simulink model "GILBERT1FINAL"  (R2023a)
settings: Solver=VariableStepAuto  StartTime=0.0  StopTime=10.0  RelTol=1e-3
undefined symbols (not defined in the file): Acid, Lead
libraries: spsSeriesRLCBranchLib x5, spsBreakerLib x4, spsBatteryLib x3, spsPVArrayLib x1, spsParallelRLCBranchLib x1, spspowerguiLib x1
settings Model: Creator=InnoTech  LastModifiedBy=Karim

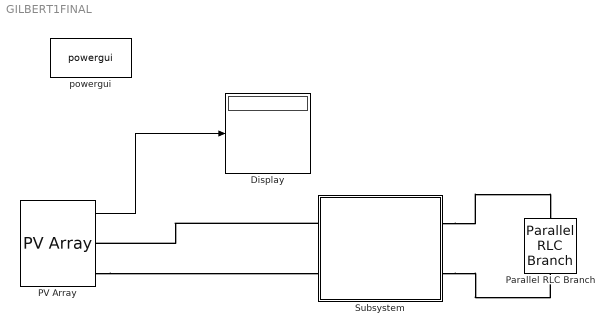
== system GILBERT1FINAL ==
  Display : Display
  PV Array : spsPVArrayLib/PV Array  Npar=40  Nser=10  PlotType=array @ 1000 W/m2 & specified temperatures  S_vec="[ 1000  500  100 ]"  Temp_C_vec="[ 45 25  ]"  ModuleName=User-defined  PlotWhenSelected=off  Pm=213.15  Ncell=60  Voc=36.3  Isc=7.84  Vm=29  Im=7.35  beta_Voc_pc=-0.36099  alpha_Isc_pc=0.102  beta_Voc=-0.13104  alpha_Isc=0.0079968  IL=7.8654  I0=2.9273e-10  nI=0.98119  Rsh=313.0553  Rs=0.39381  RobustModel=off  RobustCellTemperature=313.3991  BAL=on  Tc=1e-6  Tfilter=5e-5
  Parallel RLC Branch : spsParallelRLCBranchLib/Parallel RLC Branch  LConnTagsString=a  RConnTagsString=__new0  BranchType=RLC  Resistance=1  Inductance=1e-3  SetiL0=off  InitialCurrent=0  Capacitance=1e-6  Setx0=off  InitialVoltage=0  Measurements=None
  Subsystem : Subsystem
  powergui : spspowerguiLib/powergui  Priority=1  SimulationMode=Discrete  SampleTime=50e-6  frequency=60  Iterations=50  frequencyindice=0  Pbase=100e6  ErrMax=1e-4  UnitsV=kV  UnitsW=MW  buscounter=0  FunctionMessages=off  echomessages=off  EnableUseOfTLC=off  CurrentSourceSwitches=off  DisableSnubberDevices=off  DisableRonSwitches=off  DisableVfSwitches=off  DisplayEquations=off  AutomaticDiscreteSolvers=off  SolverType=Tustin/Backward Euler (TBE)  Interpol=off  ExternalGateDelay=off  methode=off  Ts=100  x0status=blocks  SPID=on  SwTol=0  HookPort=off  NonlinearTolerance=1e-4  nMaxIteration=100  ContinueOnMaxIteration=off  RestoreLinks=warning  ResistiveCurrentMeasurement=off  Frange=[0:2:500]  Ylog=off  Xlog=on  ShowGrid=off  save=off  variable=ZData  structure=0  ZoomFFT=off  StartTime=0.0  cycles=1  DisplayStyle=1  fundamental=60  FreqAxis=off  MaxFrequency=1000  frequencyindicesteady=1  RmsSteady=1  display=off
  wires:
  PV Array/1 -> Display/1
  connections:
  Subsystem/LConn1 -- PV Array/RConn1
  PV Array/RConn2 -- Subsystem/LConn2
  Subsystem/RConn1 -- Parallel RLC Branch/LConn1
  Subsystem/RConn2 -- Parallel RLC Branch/RConn1

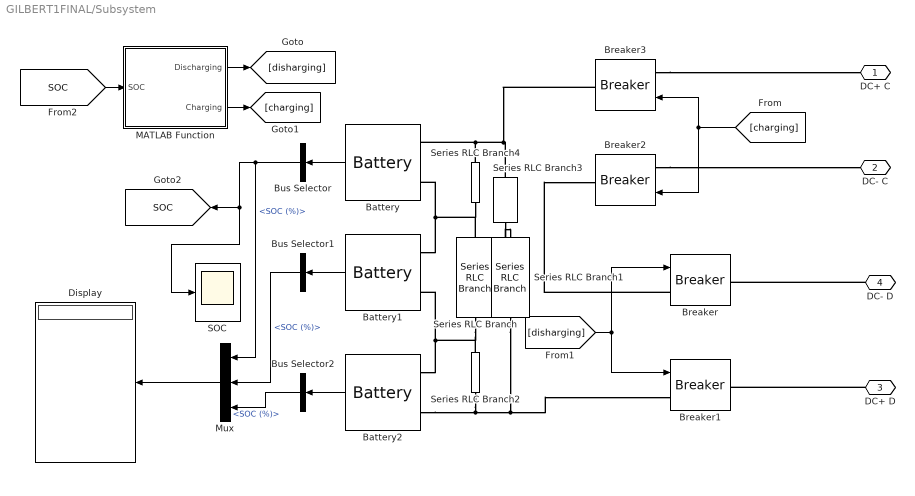
== system GILBERT1FINAL/Subsystem ==
  Battery : spsBatteryLib/Battery  BatType=Lead-Acid  NomV=12*50  NomQ=141.65  SOC=50  Batt_Tr=30  PresetModel=on  MaxQ=147.5521  MinV=450  FullV=653.2895  Dis_rate=28.33  R=0.042358  Normal_OP=43.9508  expZone="[610.8553     0.4721667]"
  Battery1 : spsBatteryLib/Battery  BatType=Lead-Acid  NomV=12*50  NomQ=141.65  SOC=50  Batt_Tr=30  PresetModel=on  MaxQ=147.5521  MinV=450  FullV=653.2895  Dis_rate=28.33  R=0.042358  Normal_OP=43.9508  expZone="[610.8553     0.4721667]"
  Battery2 : spsBatteryLib/Battery  BatType=Lead-Acid  NomV=12*50  NomQ=141.65  SOC=50  Batt_Tr=30  PresetModel=on  MaxQ=147.5521  MinV=450  FullV=653.2895  Dis_rate=28.33  R=0.042358  Normal_OP=43.9508  expZone="[610.8553     0.4721667]"
  Breaker{,1..3} (4 alike) : spsBreakerLib/Breaker  InitialState=0  SwitchingTimes="[1/60  5/60]"  External=on  BreakerResistance=0.01  SnubberResistance=1e6  SnubberCapacitance=inf  Measurements=None  MoreParameters=on  NoBreakLoop=off
  Bus Selector : BusSelector  OutputSignals=SOC (%)
  Bus Selector1 : BusSelector  OutputSignals=SOC (%)
  Bus Selector2 : BusSelector  OutputSignals=SOC (%)
  Display : Display
  MATLAB Function : MATLAB Function  TreatAsAtomicUnit=on
  Mux : Mux  Inputs=3
  SOC : Scope
  Series RLC Branch : spsSeriesRLCBranchLib/Series RLC Branch  LConnTagsString=__new0  RConnTagsString=__new0  BranchType=R  Resistance=100  Inductance=1e-3  SetiL0=off  InitialCurrent=0  Capacitance=1e-6  Setx0=off  InitialVoltage=0  Measurements=None
  Series RLC Branch1 : spsSeriesRLCBranchLib/Series RLC Branch  LConnTagsString=__new0  RConnTagsString=__new0  BranchType=C  Resistance=100  Inductance=1e-3  SetiL0=off  InitialCurrent=0  Capacitance=1e-6  Setx0=off  InitialVoltage=0  Measurements=None
  Series RLC Branch2 : spsSeriesRLCBranchLib/Series RLC Branch  LConnTagsString=__new0  RConnTagsString=__new0  BranchType=L  Resistance=100  Inductance=1e-3  SetiL0=off  InitialCurrent=0  Capacitance=1e-6  Setx0=off  InitialVoltage=0  Measurements=None
  Series RLC Branch3 : spsSeriesRLCBranchLib/Series RLC Branch  LConnTagsString=__new0  RConnTagsString=__new0  BranchType=R  Resistance=1  Inductance=1e-3  SetiL0=off  InitialCurrent=0  Capacitance=1e-6  Setx0=off  InitialVoltage=0  Measurements=None
  Series RLC Branch4 : spsSeriesRLCBranchLib/Series RLC Branch  LConnTagsString=__new0  RConnTagsString=__new0  BranchType=L  Resistance=100  Inductance=1e-3  SetiL0=off  InitialCurrent=0  Capacitance=1e-6  Setx0=off  InitialVoltage=0  Measurements=None
  DC+ C : PMIOPort  Side=Left
  DC- C : PMIOPort  Port=2  Side=Left
  DC+ D : PMIOPort  Port=3  Side=Right
  DC- D : PMIOPort  Port=4  Side=Right
  tag scope: SOC=global
  wires:
  MATLAB Function/1(Discharging) -> [disharging]
  [charging] -> Breaker2/1, Breaker3/1
  Bus Selector/1 -> Mux/1, [SOC], SOC/1  "<SOC (%)>"
  [SOC] -> MATLAB Function/1(SOC)
  MATLAB Function/2(Charging) -> [charging]
  Battery/1 -> Bus Selector/1
  [disharging] -> Breaker1/1, Breaker/1
  Battery1/1 -> Bus Selector1/1
  Bus Selector1/1 -> Mux/2  "<SOC (%)>"
  Bus Selector2/1 -> Mux/3  "<SOC (%)>"
  Battery2/1 -> Bus Selector2/1
  Mux/1 -> Display/1
  connections:
  Breaker3/RConn1 -- Series RLC Branch3/LConn1 -- Series RLC Branch4/LConn1 -- Battery/LConn1
  DC+ D/RConn1 -- Breaker1/RConn1
  Breaker2/LConn1 -- DC- C/RConn1
  DC- D/RConn1 -- Breaker/RConn1
  Breaker3/LConn1 -- DC+ C/RConn1
  Breaker/LConn1 -- Breaker2/RConn1
  Battery2/LConn2 -- Series RLC Branch2/RConn1 -- Series RLC Branch1/RConn1 -- Breaker1/LConn1
  Battery2/LConn1 -- Series RLC Branch2/LConn1 -- Series RLC Branch/RConn1 -- Battery1/LConn2
  Battery1/LConn1 -- Series RLC Branch4/RConn1 -- Series RLC Branch/LConn1 -- Battery/LConn2
  Series RLC Branch3/RConn1 -- Series RLC Branch1/LConn1

== matlab function GILBERT1FINAL/Subsystem/MATLAB Function ==
  data: Discharging output; SOC input; Charging output
function[Discharging,Charging]=CDS(SOC)
   Discharging=1;
   Charging=0;
if(SOC>=90)
   Discharging=1;
   Charging=0;
end
if(SOC<=20)
   Discharging=1;
   Charging=1;
end
